simulink subsystem "ParachuteSpatial3DOF_Force_Moment"  (R2024b)
settings: Solver=VariableStepAuto  StartTime=0.0  StopTime=10.0  RelTol=1e-3
libraries: aerolibatmos2 x1, matrix_library x1, vrlib x1
settings Model: Creator=thatf  LastModifiedBy=thatf
settings RTWCC: GPUComputeCapability=3.5

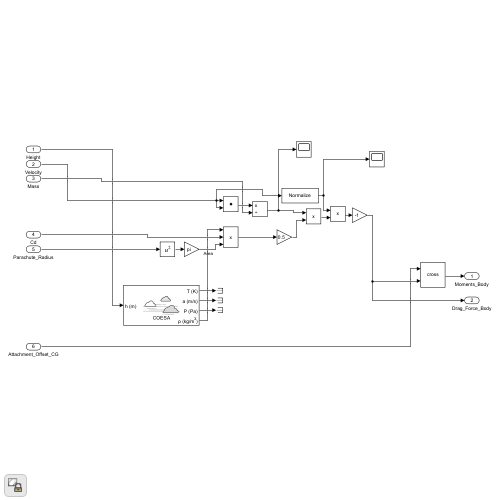
[thumbnail: Simulink's stored preview of the top-level diagram]
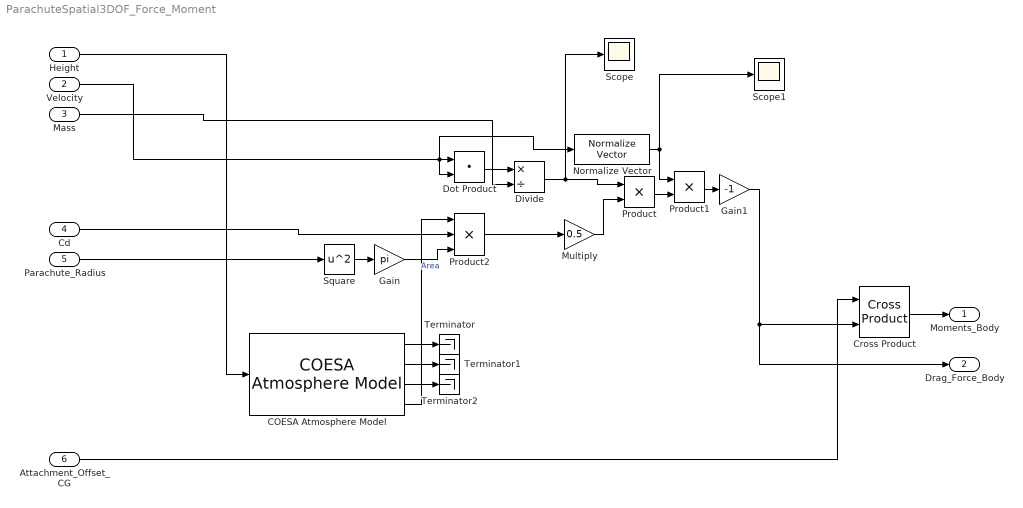
== system ParachuteSpatial3DOF_Force_Moment ==
  Height : Inport
  Velocity : Inport  Port=2
  Mass : Inport  Port=3
  Cd : Inport  Port=4
  Parachute_Radius : Inport  Port=5
  Attachment_Offset_CG : Inport  Port=6
  COESA Atmosphere Model : aerolibatmos2/COESA Atmosphere Model  units=Metric (MKS)  spec=1976 COESA-extended U.S. Standard Atmosphere  model=Profile  profile_var=High temperature  profile_percent=1%  profile_alt=5 km (16404 ft)  envelope_var=High temperature  envelope_percent=1%  action=Warning
  Cross Product : matrix_library/Cross Product
  Divide : Product  Inputs=*/
  Dot Product : DotProduct  OutDataTypeStr=Inherit: Inherit via internal rule
  Gain : Gain  Gain=pi
  Gain1 : Gain  Gain=-1
  Multiply : Gain  Gain=0.5
  Normalize Vector : vrlib/Utilities/Normalize Vector  maxzero=0
  Product : Product
  Product1 : Product
  Product2 : Product  Inputs=3
  Scope : Scope
  Scope1 : Scope
  Square : Math  Operator=square
  Terminator : Terminator
  Terminator1 : Terminator
  Terminator2 : Terminator
  Moments_Body : Outport
  Drag_Force_Body : Outport  Port=2
  wires:
  Normalize Vector/1 -> Scope1/1, Product1/1
  Divide/1 -> Product/1, Scope/1
  Product/1 -> Product1/2
  Dot Product/1 -> Divide/1
  Mass/1 -> Divide/2
  Multiply/1 -> Product/2
  Product2/1 -> Multiply/1
  Cd/1 -> Product2/2
  Square/1 -> Gain/1
  Gain/1 -> Product2/3  "Area"
  Parachute_Radius/1 -> Square/1
  COESA Atmosphere Model/4 -> Product2/1
  COESA Atmosphere Model/1 -> Terminator/1
  COESA Atmosphere Model/2 -> Terminator1/1
  COESA Atmosphere Model/3 -> Terminator2/1
  Height/1 -> COESA Atmosphere Model/1
  Product1/1 -> Gain1/1
  Attachment_Offset_CG/1 -> Cross Product/1
  Cross Product/1 -> Moments_Body/1
  Gain1/1 -> Cross Product/2, Drag_Force_Body/1
  Velocity/1 -> Dot Product/2, Dot Product/1, Normalize Vector/1
